simulink model "Full_control_with_variable_reference_velocity_2018b"  (R2018b)
settings: Solver=VariableStepAuto  StartTime=0.0  StopTime=400  RelTol=1e-3
values from neighbouring files (symbols this model uses):
  controller = optimizer(constraints, objective,[],{x{1},r,Ad_,Bd_},[u{:}])    [MPC_Script.m]
  Ka = 1/(Ki*ts/3)    (= 0.15)    [INIT.m]
  Ki = 200    [INIT.m]
  Kp = 1500    [INIT.m]
  Psi0 = 245*pi/180    (= 4.27605666739)    [INIT.m]
  Ts = 0.01    [MPC_Script.m]    (also in MPC_Sim.m)
  X0 = 0    [INIT.m]
  Y0 = 0    [INIT.m]
undefined symbols (not defined in the file or in its folder): AdaptivepurePursuitRefGen, LongDynWorking, MappingFtoW, MPC_Sim, target_acceleration, Track
libraries: simulink x5
settings Model: Creator=bensalso  LastModifiedBy=21655
settings DataIOCC: ReturnWorkspaceOutputs=on

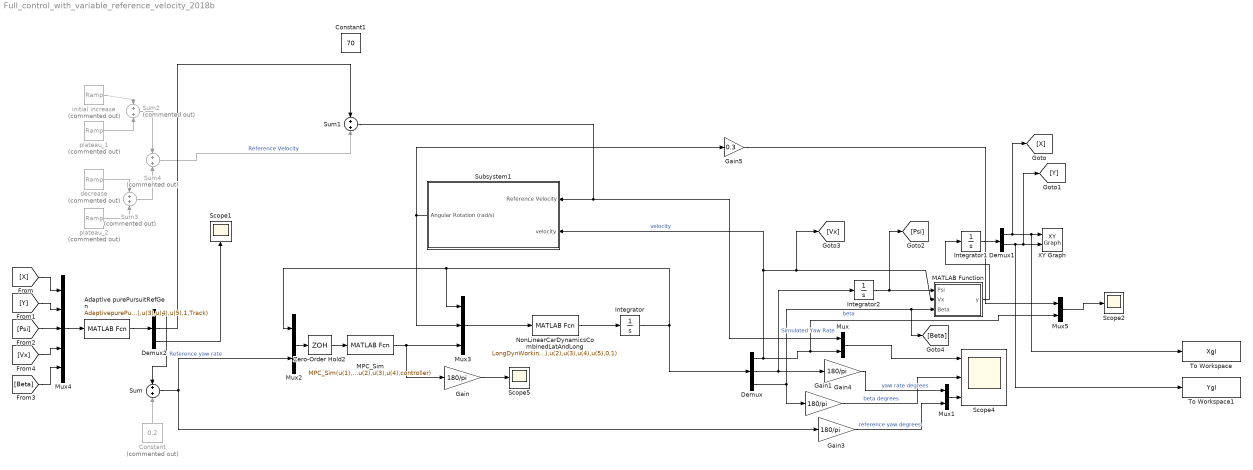
== system Full_control_with_variable_reference_velocity_2018b ==
  Adaptive purePursuitRefGen : MATLABFcn  MATLABFcn=AdaptivepurePursuitRefGen(u(1),u(2),u(3),u(4),u(5),1,Track)  OutputDimensions=3
  Constant : Constant  Commented=on  Value=0.2
  Constant1 : Constant  Value=70
  Demux : Demux  Outputs=3
  Demux1 : Demux  Outputs=2
  Demux2 : Demux  Outputs=3
  Gain{,1,3..4} (4 alike) : Gain  Gain=180/pi
  Gain5 : Gain  Gain=0.3
  Integrator : Integrator  InitialCondition=[20 ; 0; 0]
  Integrator1 : Integrator  InitialCondition=[X0, Y0]
  Integrator2 : Integrator  InitialCondition=Psi0
  MATLAB Function : MATLAB Function  TreatAsAtomicUnit=on
  MPC_Sim : MATLABFcn  MATLABFcn=MPC_Sim(u(1),u(2),u(3),u(4),controller)  OutputDimensions=1
  Mux{,1..2,5} (4 alike) : Mux  Inputs=2
  Mux3 : Mux  Inputs=3
  Mux4 : Mux  Inputs=5
  NonLinearCarDynamicsCombinedLatAndLong : MATLABFcn  MATLABFcn=LongDynWorking(u(1),u(2),u(3),u(4),u(5),0,1)  OutputDimensions=3
  Scope1 : Scope
  Scope2 : Scope
  Scope4 : Scope  NumInputPorts=3
  Scope5 : Scope
  Subsystem1 : Subsystem
  Sum : Sum
  Sum1 : Sum
  Sum2 : Sum  Commented=on
  Sum3 : Sum  Commented=on
  Sum4 : Sum  Commented=on
  To Workspace : ToWorkspace  VariableName=Xgl  SaveFormat=Timeseries  SampleTime=-1
      settings: Save2DSignal=2-D array (concatenate along first dimension)
  To Workspace1 : ToWorkspace  VariableName=Ygl  SaveFormat=Timeseries  SampleTime=-1
      settings: Save2DSignal=2-D array (concatenate along first dimension)
  XY Graph : simulink/Sinks/XY Graph  xmin=-1000  xmax=1000  ymin=-1000  ymax=1000  st=-1
  Zero-Order Hold2 : ZeroOrderHold  SampleTime=Ts
  decrease : simulink/Sources/Ramp  Commented=on  slope=-target_acceleration  start=40  InitialOutput=0
  initial increase : simulink/Sources/Ramp  Commented=on  slope=target_acceleration  start=0  InitialOutput=0
  plateau_1 : simulink/Sources/Ramp  Commented=on  slope=-target_acceleration  start=25  InitialOutput=0
  plateau_2 : simulink/Sources/Ramp  Commented=on  slope=target_acceleration  start=50  InitialOutput=0
  wires:
  Zero-Order Hold2/1 -> MPC_Sim/1
  NonLinearCarDynamicsCombinedLatAndLong/1 -> Integrator/1
  Mux2/1 -> Zero-Order Hold2/1
  Gain/1 -> Scope5/1
  Integrator/1 -> Mux2/1, Mux3/1, Demux/1
  MPC_Sim/1 -> Mux3/3, Gain/1
  Mux3/1 -> NonLinearCarDynamicsCombinedLatAndLong/1
  decrease/1 -> Sum3/1
  Sum3/1 -> Sum4/2
  plateau_2/1 -> Sum3/2
  Sum2/1 -> Sum4/1
  initial increase/1 -> Sum2/1
  plateau_1/1 -> Sum2/2
  Demux/1 -> MATLAB Function/2(Vx), [Vx], Subsystem1/2(velocity), Mux5/2, Mux/2  "velocity"
  Mux/1 -> Scope4/1
  Gain1/1 -> Scope4/2  "beta degrees"
  Gain4/1 -> Mux1/1  "yaw rate degrees"
  Gain3/1 -> Mux1/2  "reference yaw degrees"
  Mux1/1 -> Scope4/3
  Integrator1/1 -> Demux1/1
  Demux/3 -> [Beta], MATLAB Function/3(Beta), Gain1/1  "beta"
  Demux/2 -> Integrator2/1, Gain4/1  "Simulated Yaw Rate"
  MATLAB Function/1(y) -> Integrator1/1
  Subsystem1/1(Angular Rotation (rad/s)) -> Mux3/2, Gain5/1
  Sum4/1 -> Sum1/2  "Reference Velocity"
  Sum1/1 -> Mux/1, Subsystem1/1(Reference Velocity)
  Integrator2/1 -> [Psi], MATLAB Function/1(Psi)
  [X] -> Mux4/1
  [Y] -> Mux4/2
  [Psi] -> Mux4/3
  [Vx] -> Mux4/4
  [Beta] -> Mux4/5
  Mux4/1 -> Adaptive purePursuitRefGen/1
  Constant/1 -> Sum/2
  Sum/1 -> Gain3/1, Mux2/2
  Demux1/2 -> To Workspace1/1, [Y], XY Graph/2
  Demux1/1 -> [X], To Workspace/1, XY Graph/1
  Demux2/2 -> Sum1/1
  Adaptive purePursuitRefGen/1 -> Demux2/1
  Gain5/1 -> Mux5/1
  Mux5/1 -> Scope2/1
  Demux2/1 -> Sum/1  "Reference yaw rate"
  Demux2/3 -> Scope1/1

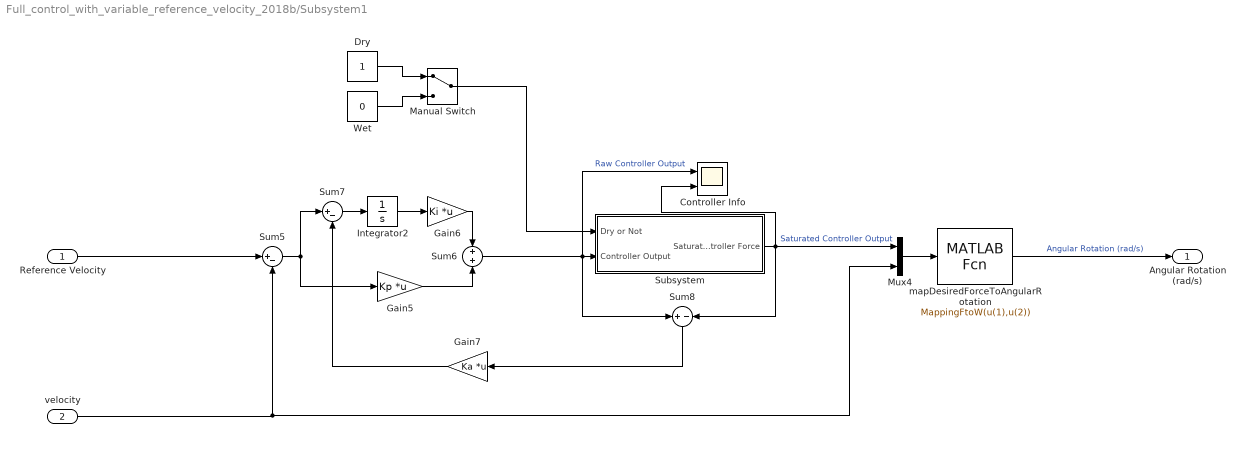
== system Full_control_with_variable_reference_velocity_2018b/Subsystem1 ==
  Reference Velocity : Inport
  velocity : Inport  Port=2
  Controller Info : Scope  NumInputPorts=2
  Dry : Constant
  Gain5 : Gain  Gain=Kp  Multiplication=Matrix(K*u)
  Gain6 : Gain  Gain=Ki  Multiplication=Matrix(K*u)
  Gain7 : Gain  Gain=Ka  Multiplication=Matrix(K*u)
  Integrator2 : Integrator  InitialCondition=0.1
  Manual Switch : ManualSwitch
  Mux4 : Mux  Inputs=2
  Subsystem : Subsystem
  Sum5 : Sum  Inputs=|+-
  Sum6 : Sum
  Sum7 : Sum  Inputs=|+-
  Sum8 : Sum  Inputs=+-
  Wet : Constant  Value=0
  mapDesiredForceToAngularRotation : MATLABFcn  MATLABFcn=MappingFtoW(u(1),u(2))  OutputDimensions=1
  Angular Rotation (rad/s) : Outport  VectorParamsAs1DForOutWhenUnconnected=off
  wires:
  Mux4/1 -> mapDesiredForceToAngularRotation/1
  Subsystem/1(Saturated Controller Force) -> Mux4/1, Controller Info/2, Sum8/2  "Saturated Controller Output"
  Gain5/1 -> Sum6/2
  Wet/1 -> Manual Switch/2
  Sum6/1 -> Controller Info/1, Sum8/1, Subsystem/2(Controller Output)  "Raw Controller Output"
  Dry/1 -> Manual Switch/1
  Integrator2/1 -> Gain6/1
  Gain7/1 -> Sum7/2
  Manual Switch/1 -> Subsystem/1(Dry or Not)
  Sum8/1 -> Gain7/1
  Gain6/1 -> Sum6/1
  velocity/1 -> Mux4/2, Sum5/2
  Sum5/1 -> Sum7/1, Gain5/1
  Sum7/1 -> Integrator2/1
  mapDesiredForceToAngularRotation/1 -> Angular Rotation (rad/s)/1  "Angular Rotation (rad/s)"
  Reference Velocity/1 -> Sum5/1

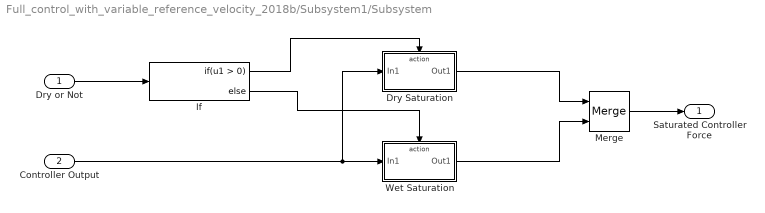
== system Full_control_with_variable_reference_velocity_2018b/Subsystem1/Subsystem ==
  Dry or Not : Inport
  Controller Output : Inport  Port=2
  Dry Saturation : Subsystem  TreatAsAtomicUnit=on
  If : If
  Merge : Merge  InitialOutput=[0]
  Wet Saturation : Subsystem  TreatAsAtomicUnit=on
  Saturated Controller Force : Outport  VectorParamsAs1DForOutWhenUnconnected=off
  wires:
  Wet Saturation/1(Out1) -> Merge/2
  Merge/1 -> Saturated Controller Force/1
  Controller Output/1 -> Dry Saturation/1(In1), Wet Saturation/1(In1)
  Dry Saturation/1(Out1) -> Merge/1
  If/1 -> Dry Saturation/Action
  Dry or Not/1 -> If/1
  If/2 -> Wet Saturation/Action

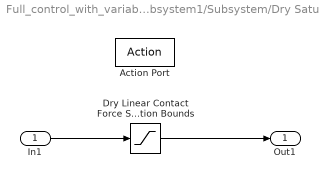
== system Full_control_with_variable_reference_velocity_2018b/Subsystem1/Subsystem/Dry Saturation ==
  In1 : Inport
  Action Port : ActionPort
  Dry Linear Contact Force Saturation Bounds : Saturate  UpperLimit=9000  LowerLimit=-9000
  Out1 : Outport  VectorParamsAs1DForOutWhenUnconnected=off
  wires:
  In1/1 -> Dry Linear Contact Force Saturation Bounds/1
  Dry Linear Contact Force Saturation Bounds/1 -> Out1/1

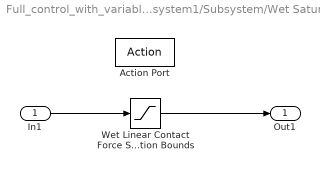
== system Full_control_with_variable_reference_velocity_2018b/Subsystem1/Subsystem/Wet Saturation ==
  In1 : Inport
  Action Port : ActionPort
  Wet Linear Contact Force Saturation Bounds : Saturate  UpperLimit=5000  LowerLimit=-5000
  Out1 : Outport  VectorParamsAs1DForOutWhenUnconnected=off
  wires:
  In1/1 -> Wet Linear Contact Force Saturation Bounds/1
  Wet Linear Contact Force Saturation Bounds/1 -> Out1/1

== matlab function Full_control_with_variable_reference_velocity_2018b/MATLAB Function ==
  data: Psi input; y output; Vx input; Beta input
function y = fcn(Psi, Vx, Beta)
    Vy = Beta*Vx;
    V = sqrt(Vx^2 + Vy^2);
    
    Xdot = V*cos(Psi+Beta);
    Ydot = V*sin(Psi+Beta);
    
    y = [Xdot, Ydot];
end
